simulink model "sm_3d_printer"  (R2023a)
settings: Solver=FixedStepAuto  StartTime=0.0  StopTime=inf  FixedStep=0.005  RelTol=1e-3
model workspace: external: MATLAB File sm_3d_printer_parameters.m (data not in the file)
undefined symbols (not defined in the file or in its folder): smiData, X, Y, Z
libraries: sm_lib x33, fl_lib x15, nesl_utility x10, ee_lib x3, slpidlib x3
(part 3 of 3)

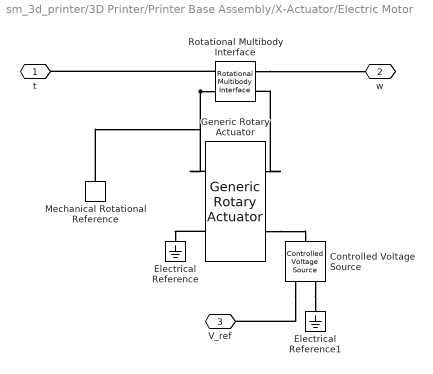
== system sm_3d_printer/3D Printer/Printer Base Assembly/X-Actuator/Electric Motor ==
  Controlled Voltage Source : fl_lib/Electrical/Electrical Sources/Controlled Voltage Source
  Electrical Reference : fl_lib/Electrical/Electrical Elements/Electrical Reference
  Electrical Reference1 : fl_lib/Electrical/Electrical Elements/Electrical Reference
  Generic Rotary Actuator : ee_lib/Electromechanical/Mechatronic Actuators/Generic Rotary Actuator  w_vec=w_m rpm  T_vec=t_m N*m  Vrated=12 V  eff=80  w_eff=2000 rpm  Pbase=0.1 W  pwm_or_av=ee.enum.pwm_or_av.pwm  J=0.1 kg*m^2  lam=1e-6 N*m/(rad/s)  i_specify=off  i_priority=None  i=0 A  i_nominal_specify=off  i_nominal_unit=A  i_nominal_value=1  t_specify=off  t_priority=None  t=0 N*m  t_nominal_specify=off  t_nominal_unit=N*m  t_nominal_value=1  w_specify=off  w_priority=None  w=0 rpm  w_nominal_specify=off  w_nominal_unit=rpm  w_nominal_value=1  alpha=3.93e-3 1/K  Tmeas=25 degC  thermal_mass=100 J/K  Q_specify=off  Q_priority=None  Q=0 W  Q_nominal_specify=off  Q_nominal_unit=W  Q_nominal_value=1  temperature_specify=off  temperature_priority=High  temperature=300 K  temperature_nominal_specify=off  temperature_nominal_unit=K  temperature_nominal_value=1
      settings: InternalSimscapePortConfiguration="{\"Bottom\":[],\"Left\":[{\"id\":\"p\",\"label\":\"+\",\"type\":\"foundation.electrical.electrical\"},{\"id\":\"R\",\"label\":\"R\",\"type\":\"foundation.mechanical.rotational.rotational\"}],\"Right\":[{\"id\":\"n\",\"label\":\"-\",\"type\":\"foundation.electrical.electrical\"},{\"id\":\"C\",\"label\":\"C\",\"type\":\"foundation.mechanical.rotational.rotational\"}],\"Top\":[]}"
  Mechanical Rotational Reference : fl_lib/Mechanical/Rotational Elements/Mechanical Rotational Reference
  Rotational Multibody Interface : fl_lib/Mechanical/Multibody Interfaces/Rotational Multibody Interface
  t : PMIOPort  Side=Left
  w : PMIOPort  Port=2  Side=Right
  V_ref : PMIOPort  Port=3  Side=Right
  connections:
  Controlled Voltage Source/RConn1 -- V_ref/RConn1
  Generic Rotary Actuator/LConn2 -- Rotational Multibody Interface/RConn2
  Controlled Voltage Source/RConn2 -- Electrical Reference1/LConn1
  Rotational Multibody Interface/LConn2 -- Mechanical Rotational Reference/LConn1 -- Generic Rotary Actuator/RConn2
  Generic Rotary Actuator/RConn1 -- Electrical Reference/LConn1
  Rotational Multibody Interface/LConn1 -- t/RConn1
  Rotational Multibody Interface/RConn1 -- w/RConn1
  Generic Rotary Actuator/LConn1 -- Controlled Voltage Source/LConn1

== system sm_3d_printer/3D Printer/Printer Base Assembly/X-Actuator/Motor ==
  Solid : sm_lib/Body Elements/File Solid  ExtGeomFileName=Motor.STEP  UnitType=FromFile  ExtGeomFileUnits=m  StepReaderType=HEX  ExportConvexHullGeometry=off  InertiaType=CalculateFromGeometry  Mass=smiData.Solid(11).mass  MassUnits=kg  CenterOfMass=smiData.Solid(11).CoM  CenterOfMassUnits=m  MomentsOfInertia=smiData.Solid(11).MoI  MomentsOfInertiaUnits=kg*m^2  ProductsOfInertia=smiData.Solid(11).PoI  ProductsOfInertiaUnits=kg*m^2  BasedOnType=Density  Density=1000  DensityUnits=kg/m^3  DoExposeReferenceFrame=off  SerializedFrames=<Frames><Frame><Id>Frame1</Id><Value><Name>CP</Name><Origin><Source>GeometricFeature</Source><FeatureName>circular curve 82</FeatureName></Origin><PrimaryAxis><DefinedDirection>+Z</DefinedDirection><Source>ReferenceFrame</Source><SourceDirection>-Z</SourceDirection><FeatureName></FeatureName></PrimaryAxis><SecondaryAxis><DefinedDirection>+X</DefinedDirection><Source>ReferenceFrame</Source><SourceDirection>+Y</SourceDirection><FeatureName></FeatureName></SecondaryAxis></Value></Frame></Frames>  GraphicType=FromGeometry  MarkerShape=Sphere  MarkerSize=10  GraphicVisPropType=SimpleVisualProperties  GraphicDiffuseColor=[0.0 0.6 0.2]  GraphicSpecularColor=[0.5 0.5 0.5 1.0]  GraphicAmbientColor=[0.15 0.15 0.15 1.0]  GraphicEmissiveColor=[0.0 0.0 0.0 1.0]  GraphicShininess=75  GraphicOpacity=smiData.Solid(11).opacity
  CP : PMIOPort  Side=Left
  connections:
  CP/RConn1 -- Solid/LConn1

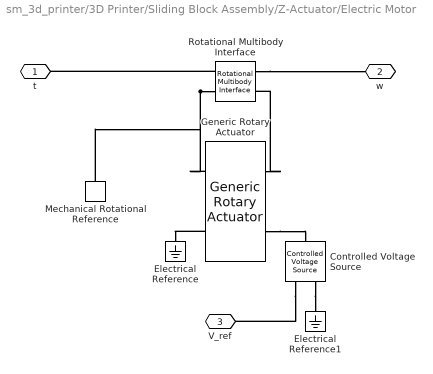
== system sm_3d_printer/3D Printer/Sliding Block Assembly/Z-Actuator/Electric Motor ==
  Controlled Voltage Source : fl_lib/Electrical/Electrical Sources/Controlled Voltage Source
  Electrical Reference : fl_lib/Electrical/Electrical Elements/Electrical Reference
  Electrical Reference1 : fl_lib/Electrical/Electrical Elements/Electrical Reference
  Generic Rotary Actuator : ee_lib/Electromechanical/Mechatronic Actuators/Generic Rotary Actuator  w_vec=w_m rpm  T_vec=t_m N*m  Vrated=12 V  eff=80  w_eff=2000 rpm  Pbase=0.1 W  pwm_or_av=ee.enum.pwm_or_av.pwm  J=0.1 kg*m^2  lam=1e-6 N*m/(rad/s)  i_specify=off  i_priority=None  i=0 A  i_nominal_specify=off  i_nominal_unit=A  i_nominal_value=1  t_specify=off  t_priority=None  t=0 N*m  t_nominal_specify=off  t_nominal_unit=N*m  t_nominal_value=1  w_specify=off  w_priority=None  w=0 rpm  w_nominal_specify=off  w_nominal_unit=rpm  w_nominal_value=1  alpha=3.93e-3 1/K  Tmeas=25 degC  thermal_mass=100 J/K  Q_specify=off  Q_priority=None  Q=0 W  Q_nominal_specify=off  Q_nominal_unit=W  Q_nominal_value=1  temperature_specify=off  temperature_priority=High  temperature=300 K  temperature_nominal_specify=off  temperature_nominal_unit=K  temperature_nominal_value=1
      settings: InternalSimscapePortConfiguration="{\"Bottom\":[],\"Left\":[{\"id\":\"p\",\"label\":\"+\",\"type\":\"foundation.electrical.electrical\"},{\"id\":\"R\",\"label\":\"R\",\"type\":\"foundation.mechanical.rotational.rotational\"}],\"Right\":[{\"id\":\"n\",\"label\":\"-\",\"type\":\"foundation.electrical.electrical\"},{\"id\":\"C\",\"label\":\"C\",\"type\":\"foundation.mechanical.rotational.rotational\"}],\"Top\":[]}"
  Mechanical Rotational Reference : fl_lib/Mechanical/Rotational Elements/Mechanical Rotational Reference
  Rotational Multibody Interface : fl_lib/Mechanical/Multibody Interfaces/Rotational Multibody Interface
  t : PMIOPort  Side=Left
  w : PMIOPort  Port=2  Side=Right
  V_ref : PMIOPort  Port=3  Side=Right
  connections:
  Controlled Voltage Source/RConn1 -- V_ref/RConn1
  Generic Rotary Actuator/LConn2 -- Rotational Multibody Interface/RConn2
  Controlled Voltage Source/RConn2 -- Electrical Reference1/LConn1
  Rotational Multibody Interface/LConn2 -- Mechanical Rotational Reference/LConn1 -- Generic Rotary Actuator/RConn2
  Generic Rotary Actuator/RConn1 -- Electrical Reference/LConn1
  Rotational Multibody Interface/LConn1 -- t/RConn1
  Rotational Multibody Interface/RConn1 -- w/RConn1
  Generic Rotary Actuator/LConn1 -- Controlled Voltage Source/LConn1

== system sm_3d_printer/3D Printer/Sliding Block Assembly/Z-Actuator/Motor ==
  Solid : sm_lib/Body Elements/File Solid  ExtGeomFileName=Motor.STEP  UnitType=FromFile  ExtGeomFileUnits=m  StepReaderType=HEX  ExportConvexHullGeometry=off  InertiaType=CalculateFromGeometry  Mass=smiData.Solid(11).mass  MassUnits=kg  CenterOfMass=smiData.Solid(11).CoM  CenterOfMassUnits=m  MomentsOfInertia=smiData.Solid(11).MoI  MomentsOfInertiaUnits=kg*m^2  ProductsOfInertia=smiData.Solid(11).PoI  ProductsOfInertiaUnits=kg*m^2  BasedOnType=Density  Density=1000  DensityUnits=kg/m^3  DoExposeReferenceFrame=off  SerializedFrames=<Frames><Frame><Id>Frame1</Id><Value><Name>CP</Name><Origin><Source>GeometricFeature</Source><FeatureName>circular curve 82</FeatureName></Origin><PrimaryAxis><DefinedDirection>+Z</DefinedDirection><Source>ReferenceFrame</Source><SourceDirection>-Z</SourceDirection><FeatureName></FeatureName></PrimaryAxis><SecondaryAxis><DefinedDirection>+X</DefinedDirection><Source>ReferenceFrame</Source><SourceDirection>+Y</SourceDirection><FeatureName></FeatureName></SecondaryAxis></Value></Frame></Frames>  GraphicType=FromGeometry  MarkerShape=Sphere  MarkerSize=10  GraphicVisPropType=SimpleVisualProperties  GraphicDiffuseColor=[0.0 0.6 0.2]  GraphicSpecularColor=[0.5 0.5 0.5 1.0]  GraphicAmbientColor=[0.15 0.15 0.15 1.0]  GraphicEmissiveColor=[0.0 0.0 0.0 1.0]  GraphicShininess=75  GraphicOpacity=smiData.Solid(11).opacity
  CP : PMIOPort  Side=Left
  connections:
  CP/RConn1 -- Solid/LConn1

== matlab function sm_3d_printer/3D Printer/MATLAB Function ==
  settings: updateMethod=DISCRETE
  data: x output; set_point input; y output; is_rapid input; position input; velocity input; prev_setpoint input; z output; norm_pos_error output; out_position output; reached output; out_set_point output
function [x,y,z,norm_pos_error,out_position,reached,out_set_point] = ParseMessages(set_point, is_rapid, position, velocity, prev_setpoint)
    
    % Set-point pass through
    x = set_point(1);
    y = set_point(2);
    z = set_point(3);
    % Position pass through
    out_position   = position;
    reached        = false; % is setpoint reached
    norm_pos_error = 0;     % norm of position error

    persistent is_new_setpoint;
    if isempty(is_new_setpoint)
        is_new_setpoint=true;
    end
    
    % % Counter
    % persistent i;
    % if isempty(i)
    %     i=0;
    % end

    % Check if there's a new setpoint
    if ~isequal(set_point,prev_setpoint)
        is_new_setpoint = true;
        % fprintf("New setpoint\n")
    end
    out_set_point = set_point;

   % If there's a rapid request
    if is_rapid == true
        norm_pos_error = norm(set_point - position);
        norm_velocity  = norm(velocity);
        
        if norm_pos_error < 0.01 & norm_velocity < 0.01 & is_new_setpoint
            reached = true;
            % fprintf("-------- %f --------\n", i);
            % fprintf("Position error: %f [mm]\n", norm_pos_error);
            % fprintf("Speed         : %f [mm/s]\n", norm_velocity);
            % i=i+1;
            is_new_setpoint = false;
        end
    end
